simulink model "simu_final_velocidade"  (R2018b)
settings: Solver=FixedStepAuto  StartTime=0.0  StopTime=2.5  FixedStep=0.001  RelTol=1e-3
values from neighbouring files (symbols this model uses):
  G = tf(c1,[1 c2])    [calculos2.m]    (also in calculos_mf.m = c1/(s+c2))
  Ki = wn^2/c1    [calculos2.m]
  Kp = (2*zeta*wn - c2)/c1    [calculos2.m]
undefined symbols (not defined in the file or in its folder): DiscIntNeverNeededParam
settings Model: Creator=lubuntu  LastModifiedBy=lubuntu

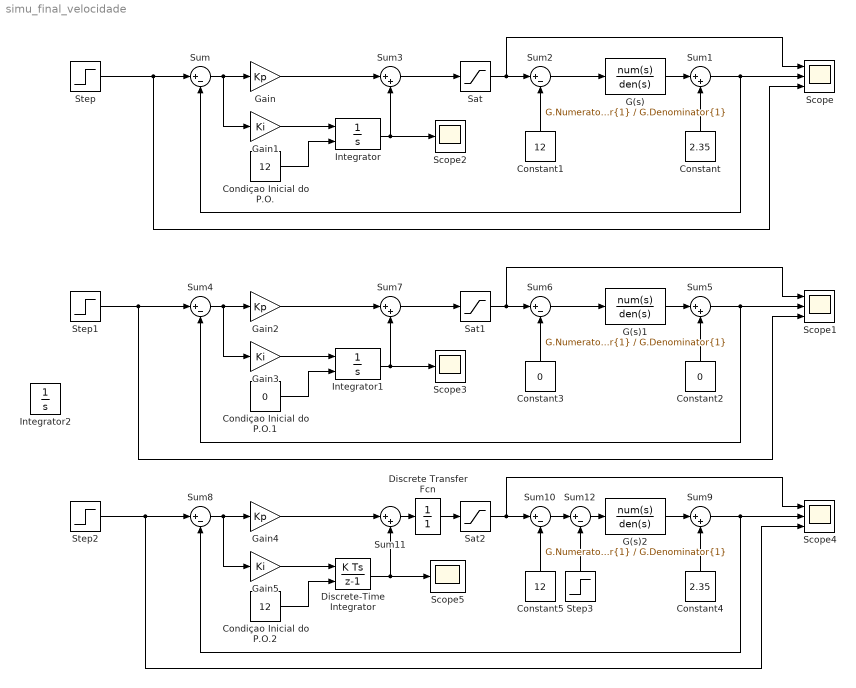
== system simu_final_velocidade ==
  Condiçao Inicial do P.O. : Constant  Value=12
  Condiçao Inicial do P.O.1 : Constant  Value=0
  Condiçao Inicial do P.O.2 : Constant  Value=12
  Constant : Constant  Value=2.35
  Constant1 : Constant  Value=12
  Constant2 : Constant  Value=0
  Constant3 : Constant  Value=0
  Constant4 : Constant  Value=2.35
  Constant5 : Constant  Value=12
  Discrete Transfer Fcn : DiscreteTransferFcn  Denominator=[1]  SampleTime=0.05
  Discrete-Time Integrator : DiscreteIntegrator  InitialConditionSource=external  InitialCondition=12  SampleTime=0.05  LimitOutput=on  UpperSaturationLimit=24  LowerSaturationLimit=-24  ICPrevOutput=DiscIntNeverNeededParam  ICPrevScaledInput=DiscIntNeverNeededParam
  G(s) : TransferFcn  Numerator=G.Numerator{1}  Denominator=G.Denominator{1}
  G(s)1 : TransferFcn  Numerator=G.Numerator{1}  Denominator=G.Denominator{1}
  G(s)2 : TransferFcn  Numerator=G.Numerator{1}  Denominator=G.Denominator{1}
  Gain : Gain  Gain=Kp
  Gain1 : Gain  Gain=Ki
  Gain2 : Gain  Gain=Kp
  Gain3 : Gain  Gain=Ki
  Gain4 : Gain  Gain=Kp
  Gain5 : Gain  Gain=Ki
  Integrator : Integrator  InitialConditionSource=external  LimitOutput=on  UpperSaturationLimit=24  LowerSaturationLimit=-24
  Integrator1 : Integrator  InitialConditionSource=external  LimitOutput=on  UpperSaturationLimit=24  LowerSaturationLimit=-24
  Integrator2 : Integrator  InitialConditionSource=external  LimitOutput=on  UpperSaturationLimit=24  LowerSaturationLimit=-24
  Sat : Saturate  UpperLimit=24  LowerLimit=0
  Sat1 : Saturate  UpperLimit=24  LowerLimit=0
  Sat2 : Saturate  UpperLimit=24  LowerLimit=0
  Scope : Scope  NumInputPorts=3
  Scope1 : Scope  NumInputPorts=3
  Scope2 : Scope
  Scope3 : Scope
  Scope4 : Scope  NumInputPorts=3
  Scope5 : Scope
  Step : Step  Time=0  After=2.59  SampleTime=0
  Step1 : Step  Time=0  After=2.35  SampleTime=0
  Step2 : Step  Time=0  After=2.35  SampleTime=0
  Step3 : Step  After=5  SampleTime=0
  Sum{,2,4,6,8,10,12} (7 alike) : Sum  Inputs=|+-
  Sum{1,3,5,7,9,11} (6 alike) : Sum  Inputs=|++
  wires:
  Sat/1 -> Sum2/1, Scope/1
  Sum1/1 -> Scope/2, Sum/2
  Step/1 -> Scope/3, Sum/1
  G(s)/1 -> Sum1/1
  Constant/1 -> Sum1/2
  Sum2/1 -> G(s)/1
  Constant1/1 -> Sum2/2
  Sum/1 -> Gain1/1, Gain/1
  Gain/1 -> Sum3/1
  Sum3/1 -> Sat/1
  Gain1/1 -> Integrator/1
  Integrator/1 -> Scope2/1, Sum3/2
  Condiçao Inicial do P.O./1 -> Integrator/2
  Constant2/1 -> Sum5/2
  Sum4/1 -> Gain3/1, Gain2/1
  Sum5/1 -> Scope1/2, Sum4/2
  Gain2/1 -> Sum7/1
  Sum7/1 -> Sat1/1
  G(s)1/1 -> Sum5/1
  Constant3/1 -> Sum6/2
  Step1/1 -> Scope1/3, Sum4/1
  Condiçao Inicial do P.O.1/1 -> Integrator1/2
  Integrator1/1 -> Scope3/1, Sum7/2
  Gain3/1 -> Integrator1/1
  Sum6/1 -> G(s)1/1
  Sat1/1 -> Sum6/1, Scope1/1
  Constant4/1 -> Sum9/2
  Sum8/1 -> Gain5/1, Gain4/1
  Sum9/1 -> Scope4/2, Sum8/2
  Gain4/1 -> Sum11/1
  G(s)2/1 -> Sum9/1
  Constant5/1 -> Sum10/2
  Step2/1 -> Scope4/3, Sum8/1
  Condiçao Inicial do P.O.2/1 -> Discrete-Time Integrator/2
  Discrete-Time Integrator/1 -> Scope5/1, Sum11/2
  Gain5/1 -> Discrete-Time Integrator/1
  Sat2/1 -> Sum10/1, Scope4/1
  Sum10/1 -> Sum12/1
  Sum12/1 -> G(s)2/1
  Step3/1 -> Sum12/2
  Sum11/1 -> Discrete Transfer Fcn/1
  Discrete Transfer Fcn/1 -> Sat2/1
